simulink model "EduRover_balance"  (R2018b)
settings: Solver=VariableStepAuto  StartTime=0.0  StopTime=10.0  RelTol=1e-3
values from neighbouring files (symbols this model uses):
  A1 = [ ... (first row only)    [parameters.m]
  a_r = 0.996    [parameters.m]
  B1 = [ ... (first row only)    [parameters.m]
  C1 = eye(4)    [parameters.m]
  D1 = zeros(4, 2)    [parameters.m]
  k_f = KK(1, 1:4)    [parameters.m]
  k_i = KK(1, 5)    [parameters.m]
  ts1 = 0.002    [parameters.m]
settings Model: Creator=CHEI  LastModifiedBy=CHEI

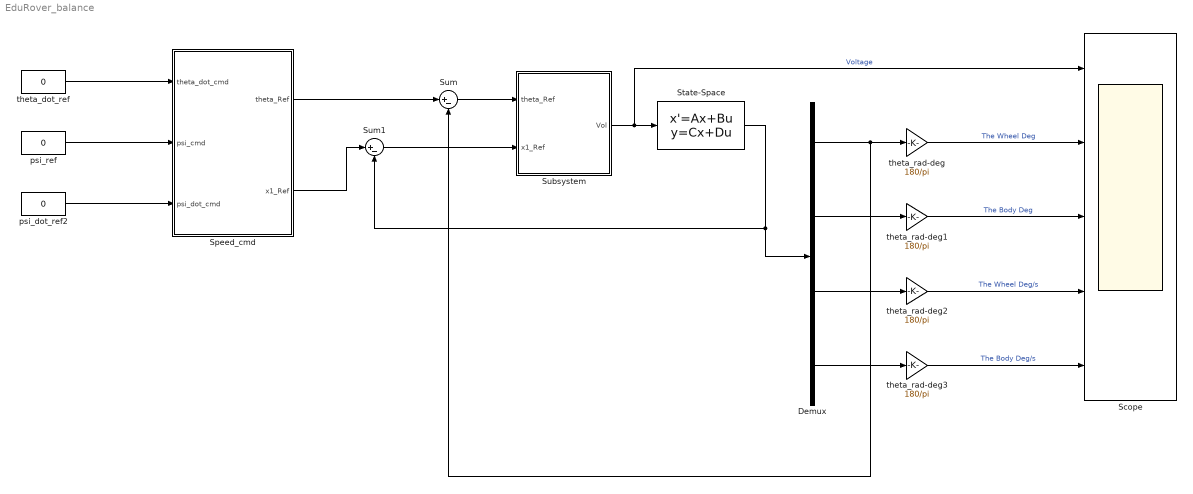
== system EduRover_balance ==
  Demux : Demux
  Scope : Scope  NumInputPorts=5
  Speed_cmd : Subsystem
  State-Space : StateSpace  A=A1  B=B1  C=C1  D=D1  InitialCondition=[0.1;5*pi/180;0;0]
  Subsystem : Subsystem
  Sum : Sum  Inputs=|+-
  Sum1 : Sum  Inputs=|+-
  psi_dot_ref2 : Constant  Value=0
  psi_ref : Constant  Value=0
  theta_dot_ref : Constant  Value=0
  theta_rad-deg{,1..3} (4 alike) : Gain  Gain=180/pi  SaturateOnIntegerOverflow=on  OutDataTypeStr=Inherit: Same as input  ParamDataTypeStr=Inherit: Same as input
  wires:
  theta_dot_ref/1 -> Speed_cmd/1(theta_dot_cmd)
  psi_ref/1 -> Speed_cmd/2(psi_cmd)
  psi_dot_ref2/1 -> Speed_cmd/3(psi_dot_cmd)
  Speed_cmd/1(theta_Ref) -> Sum/1
  Sum/1 -> Subsystem/1(theta_Ref)
  Sum1/1 -> Subsystem/2(x1_Ref)
  Speed_cmd/2(x1_Ref) -> Sum1/1
  State-Space/1 -> Sum1/2, Demux/1
  Demux/1 -> Sum/2, theta_rad-deg/1
  Demux/2 -> theta_rad-deg1/1
  Demux/3 -> theta_rad-deg2/1
  Demux/4 -> theta_rad-deg3/1
  theta_rad-deg/1 -> Scope/2  "The Wheel Deg"
  theta_rad-deg1/1 -> Scope/3  "The Body Deg"
  theta_rad-deg2/1 -> Scope/4  "The Wheel Deg/s"
  theta_rad-deg3/1 -> Scope/5  "The Body Deg/s"
  Subsystem/1(Vol) -> Scope/1, State-Space/1  "Voltage"

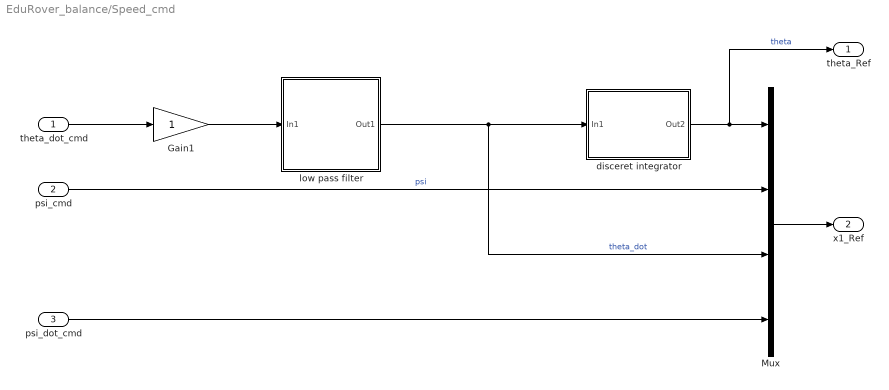
== system EduRover_balance/Speed_cmd ==
  theta_dot_cmd : Inport
  psi_cmd : Inport  Port=2
  psi_dot_cmd : Inport  Port=3
  Gain1 : Gain  OutDataTypeStr=Inherit: Same as input  ParamDataTypeStr=Inherit: Same as input
  Mux : Mux
  disceret integrator : Subsystem
  low pass filter : Subsystem
  theta_Ref : Outport
  x1_Ref : Outport  Port=2
  wires:
  low pass filter/1(Out1) -> Mux/3, disceret integrator/1(In1)  "theta_dot"
  psi_dot_cmd/1 -> Mux/4
  theta_dot_cmd/1 -> Gain1/1
  psi_cmd/1 -> Mux/2  "psi"
  disceret integrator/1(Out2) -> theta_Ref/1, Mux/1  "theta"
  Mux/1 -> x1_Ref/1
  Gain1/1 -> low pass filter/1(In1)

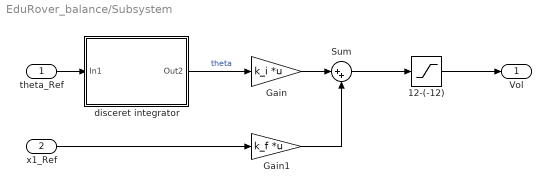
== system EduRover_balance/Subsystem ==
  theta_Ref : Inport
  x1_Ref : Inport  Port=2
  12-(-12) : Saturate  UpperLimit=12  LowerLimit=-12
  Gain : Gain  Gain=k_i  Multiplication=Matrix(K*u)
  Gain1 : Gain  Gain=k_f  Multiplication=Matrix(K*u)
  Sum : Sum  Inputs=|++  OutDataTypeStr=Inherit: Same as first input
  disceret integrator : Subsystem
  Vol : Outport
  wires:
  Sum/1 -> 12-(-12)/1
  Gain1/1 -> Sum/2
  12-(-12)/1 -> Vol/1
  theta_Ref/1 -> disceret integrator/1(In1)
  Gain/1 -> Sum/1
  disceret integrator/1(Out2) -> Gain/1  "theta"
  x1_Ref/1 -> Gain1/1

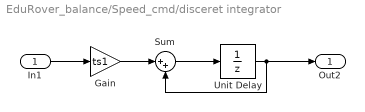
== system EduRover_balance/Speed_cmd/disceret integrator ==
  In1 : Inport
  Gain : Gain  Gain=ts1
  Sum : Sum  Inputs=|++  OutDataTypeStr=Inherit: Same as first input
  Unit Delay : UnitDelay  SampleTime=-1
  Out2 : Outport
  wires:
  Unit Delay/1 -> Out2/1, Sum/2
  In1/1 -> Gain/1
  Gain/1 -> Sum/1
  Sum/1 -> Unit Delay/1

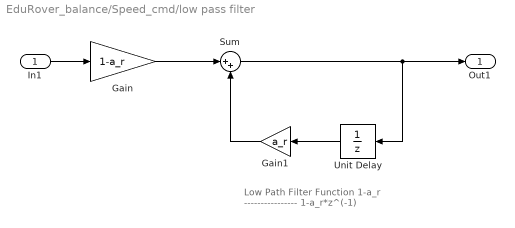
== system EduRover_balance/Speed_cmd/low pass filter ==
  note: Low Path Filter Function
      |               1-a_r
      |          ----------------
      |          1-a_r*z^(-1)
  In1 : Inport
  Gain : Gain  Gain=1-a_r
  Gain1 : Gain  Gain=a_r
  Sum : Sum  Inputs=|++  OutDataTypeStr=Inherit: Same as first input
  Unit Delay : UnitDelay  SampleTime=-1
  Out1 : Outport
  wires:
  Gain/1 -> Sum/1
  Unit Delay/1 -> Gain1/1
  In1/1 -> Gain/1
  Sum/1 -> Out1/1, Unit Delay/1
  Gain1/1 -> Sum/2

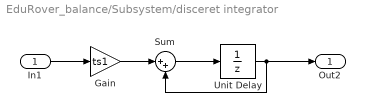
== system EduRover_balance/Subsystem/disceret integrator ==
  In1 : Inport
  Gain : Gain  Gain=ts1
  Sum : Sum  Inputs=|++  OutDataTypeStr=Inherit: Same as first input
  Unit Delay : UnitDelay  SampleTime=-1
  Out2 : Outport
  wires:
  Unit Delay/1 -> Out2/1, Sum/2
  In1/1 -> Gain/1
  Gain/1 -> Sum/1
  Sum/1 -> Unit Delay/1
